simulink model "AtomicDualRate"  (R2017a)
settings: Solver=FixedStepAuto  StartTime=0.0  StopTime=10.0  RelTol=1e-3
undefined symbols (not defined in the file): Point
libraries: robotlib x5
settings Model: Creator=marco  LastModifiedBy=marco
settings OptimizationCC: PassReuseOutputArgsAs=Individual arguments  MaxStackSize=64
settings DebuggingCC: ParameterTunabilityLossMsg=error
settings HardwareCC: ProdBitPerPointer=32  ProdBitPerSizeT=32  ProdBitPerPtrDiffT=32  ProdLargestAtomicFloat=None  ProdIntDivRoundTo=Undefined  ProdEndianess=Unspecified  ProdWordSize=32  ProdHWDeviceType=Generic->Unspecified (assume 32-bit Generic)
settings SFSimCC: MATLABDynamicMemAlloc=off
settings RTWCC: SystemTargetFile=ert.tlc  HardwareBoard=Robot Operating System (ROS)  TLCOptions="-aInlineSetEventsForThisBaseRateFcn=TLC_FALSE -aSuppressMultiTaskScheduler=TLC_FALSE  -aRateBasedStepFcn=0"  TemplateMakefile=ert_default_tmf  Description=Embedded Coder  GenerateReport=on  Toolchain=Catkin  IncludeHyperlinkInReport=on  LaunchReport=on  TargetLang=C++  GenerateTraceInfo=on  GenerateTraceReport=on  GenerateTraceReportSl=on  GenerateTraceReportSf=on  GenerateTraceReportEml=on
settings CodeAppCC: ForceParamTrailComments=on  IgnoreCustomStorageClasses=off  OperatorAnnotations=on  SimulinkDataObjDesc=on  SFDataObjDesc=on  MATLABFcnDesc=on  InsertBlockDesc=on  MATLABSourceComments=on
settings ERTTargetCC: SupportContinuousTime=on

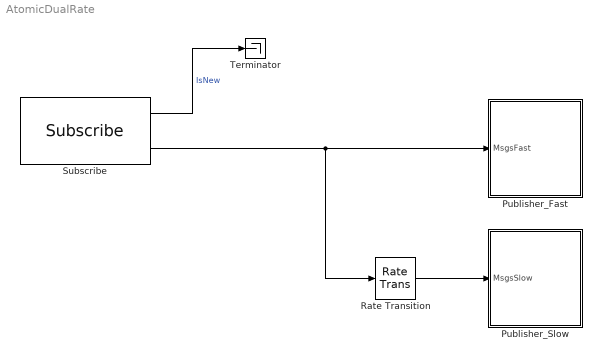
== system AtomicDualRate ==
  Publisher_Fast : Subsystem  TreatAsAtomicUnit=on  SystemSampleTime=0.01
  Publisher_Slow : Subsystem  TreatAsAtomicUnit=on  SystemSampleTime=0.05
  Rate Transition : RateTransition  OutPortSampleTimeOpt=Inherit
  Subscribe : robotlib/Subscribe  SourceLibraryInfo=This block requires Robotics System Toolbox  topicSource=Specify your own  topic=/chatter  messageType=geometry_msgs/PoseArray  sampleTime=-1  messageQueueLength=1
      settings: SourceProductBaseCode=RO
  Terminator : Terminator
  wires:
  Subscribe/1 -> Terminator/1  "IsNew"
  Subscribe/2 -> Rate Transition/1, Publisher_Fast/1(MsgsFast)
  Rate Transition/1 -> Publisher_Slow/1(MsgsSlow)

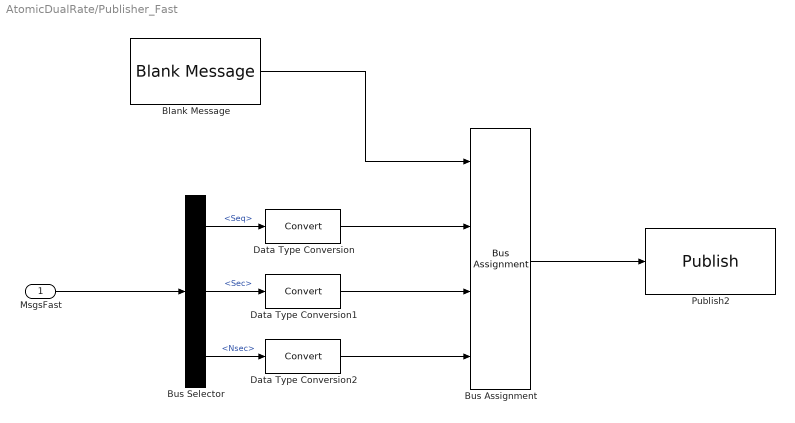
== system AtomicDualRate/Publisher_Fast ==
  MsgsFast : Inport
  Blank Message : robotlib/Blank Message  SourceLibraryInfo=This block requires Robotics System Toolbox  messageType=geometry_msgs/PointStamped  SampleTime=inf
      settings: SourceProductBaseCode=RO
  Bus Assignment : BusAssignment  AssignedSignals=Point.X,Point.Y,Point.Z
  Bus Selector : BusSelector  OutputSignals=Header.Seq,Header.Stamp.Sec,Header.Stamp.Nsec
  Data Type Conversion : DataTypeConversion
  Data Type Conversion1 : DataTypeConversion
  Data Type Conversion2 : DataTypeConversion
  Publish2 : robotlib/Publish  SourceLibraryInfo=This block requires Robotics System Toolbox  topicSource=Specify your own  topic=/Chatter_Fast  messageType=geometry_msgs/PointStamped  messageQueueLength=1
      settings: SourceProductBaseCode=RO
  wires:
  Data Type Conversion/1 -> Bus Assignment/2
  Data Type Conversion1/1 -> Bus Assignment/3
  Bus Assignment/1 -> Publish2/1
  Data Type Conversion2/1 -> Bus Assignment/4
  Blank Message/1 -> Bus Assignment/1
  Bus Selector/2 -> Data Type Conversion1/1  "<Sec>"
  Bus Selector/1 -> Data Type Conversion/1  "<Seq>"
  Bus Selector/3 -> Data Type Conversion2/1  "<Nsec>"
  MsgsFast/1 -> Bus Selector/1

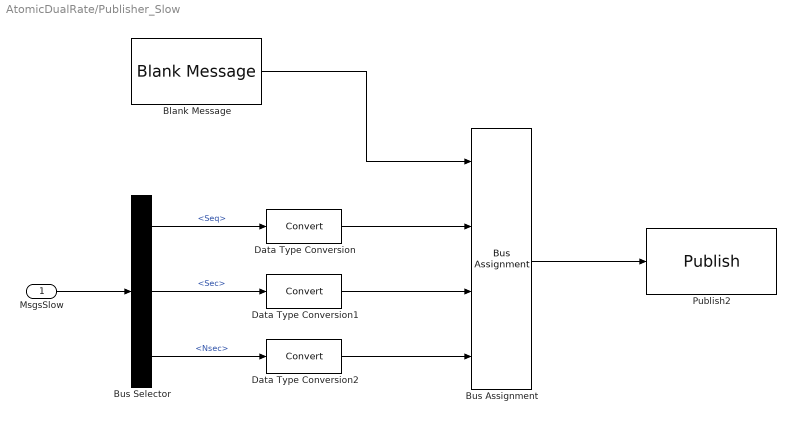
== system AtomicDualRate/Publisher_Slow ==
  MsgsSlow : Inport
  Blank Message : robotlib/Blank Message  SourceLibraryInfo=This block requires Robotics System Toolbox  messageType=geometry_msgs/PointStamped  SampleTime=inf
      settings: SourceProductBaseCode=RO
  Bus Assignment : BusAssignment  AssignedSignals=Point.X,Point.Y,Point.Z
  Bus Selector : BusSelector  OutputSignals=Header.Seq,Header.Stamp.Sec,Header.Stamp.Nsec
  Data Type Conversion : DataTypeConversion
  Data Type Conversion1 : DataTypeConversion
  Data Type Conversion2 : DataTypeConversion
  Publish2 : robotlib/Publish  SourceLibraryInfo=This block requires Robotics System Toolbox  topicSource=Specify your own  topic=/Chatter_Slow  messageType=geometry_msgs/PointStamped  messageQueueLength=1
      settings: SourceProductBaseCode=RO
  wires:
  Data Type Conversion/1 -> Bus Assignment/2
  Data Type Conversion1/1 -> Bus Assignment/3
  Bus Assignment/1 -> Publish2/1
  Data Type Conversion2/1 -> Bus Assignment/4
  Blank Message/1 -> Bus Assignment/1
  Bus Selector/2 -> Data Type Conversion1/1  "<Sec>"
  Bus Selector/1 -> Data Type Conversion/1  "<Seq>"
  Bus Selector/3 -> Data Type Conversion2/1  "<Nsec>"
  MsgsSlow/1 -> Bus Selector/1
